simulink model "P_4_3_a_Periodikus"  (R2022b)
settings: Solver=VariableStepAuto  StartTime=0.0  StopTime=10  RelTol=1e-3
undefined symbols (not defined in the file or in its folder): m, n
libraries: simulink x1
settings Model: Creator=csoka  LastModifiedBy=Mark
settings SolverCC: AlgebraicLoopSolver=TrustRegion
settings DebuggingCC: UnconnectedInputMsg=warning  UnconnectedOutputMsg=warning  UnconnectedLineMsg=warning  SFMachineParentedDataDiag=warning
settings ModelReferenceCC: EnableRefExpFcnMdlSchedulingChecks=on
settings RTWCC: DLArmComputeVersion=19.05

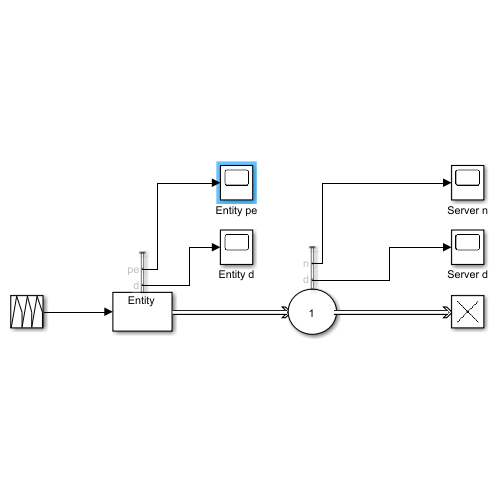
[thumbnail: Simulink's stored preview of the top-level diagram]
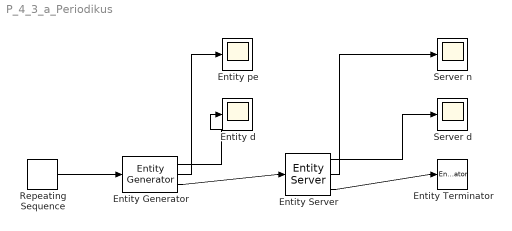
== system P_4_3_a_Periodikus ==
  Entity Generator : EntityGenerator  OutputPortMessageModes=n,n,m  TimeSource=Signal port  IntergenerationTimeAction=|  NumberEntitiesDeparted=on  PendingEntityInBlock=on  EntityType=Structured  EntityTypeName=Entity
      | persistent rngInit;
      | if isempty(rngInit)
      |     seed = 12345;
      |     rng(seed);
      |     rngInit = true;
      | end
      | 
      | % Pattern: Exponential distribution
      | mu = 1;
      | dt = -mu * log(1 - rand());
      settings: InputPortMap=u1  OutputPortMap=o0,o1,o3
  Entity Server : EntityServer  InputPortMessageModes=m  OutputPortMessageModes=n,n,m  Capacity=1  NumberEntitiesDeparted=on  NumberEntitiesInBlock=on
      settings: OutputPortMap=o0,o1,o9
  Entity Terminator : EntityTerminator  InputPortMessageModes=m
  Entity d : Scope
  Entity pe : Scope
  Repeating Sequence : simulink/Sources/Repeating Sequence  rep_seq_t=[0 1 2]  rep_seq_y=[1 3 2].'
  Server d : Scope
  Server n : Scope
  wires:
  Entity Server/3 -> Entity Terminator/1
  Entity Server/1 -> Server d/1
  Entity Server/2 -> Server n/1
  Entity Generator/1 -> Entity d/1
  Entity Generator/2 -> Entity pe/1
  Entity Generator/3 -> Entity Server/1
  Repeating Sequence/1 -> Entity Generator/1
